simulink model "saturazione"  (R2017a)
settings: Solver=VariableStepAuto  StartTime=0.0  StopTime=50  RelTol=1e-3
settings Model: Creator=Enrico Donato  LastModifiedBy=Enrico Donato

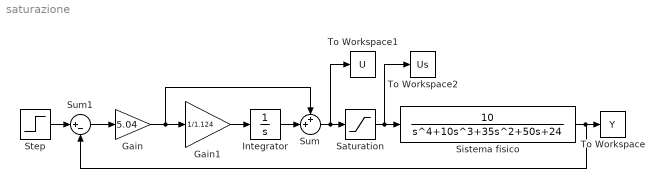
== system saturazione ==
  Gain : Gain  Gain=5.04
  Gain1 : Gain  Gain=1/1.124
  Integrator : Integrator
  Saturation : Saturate  UpperLimit=3.5  LowerLimit=-3.5
  Sistema fisico : TransferFcn  Numerator=[10]  Denominator=[1 10 35 50 24]
  Step : Step  Time=0  SampleTime=0
  Sum : Sum  Inputs=++|
  Sum1 : Sum  Inputs=|+-
  To Workspace : ToWorkspace  VariableName=Y  SampleTime=-1
  To Workspace1 : ToWorkspace  VariableName=U  SampleTime=-1
  To Workspace2 : ToWorkspace  VariableName=Us  SampleTime=-1
  wires:
  Sum/1 -> To Workspace1/1, Saturation/1
  Gain1/1 -> Integrator/1
  Integrator/1 -> Sum/2
  Sum1/1 -> Gain/1
  Gain/1 -> Sum/1, Gain1/1
  Sistema fisico/1 -> Sum1/2, To Workspace/1
  Step/1 -> Sum1/1
  Saturation/1 -> To Workspace2/1, Sistema fisico/1
